simulink model "buckcomverter+battery"  (R2020a)
settings: Solver=VariableStepAuto  StartTime=0.0  StopTime=5  RelTol=1e-3
undefined symbols (not defined in the file): Acid, Down, Lead, Up
libraries: powerlib x9, electricdrivelib x1, eePwmGenerator x1
settings Model: Creator=Asus  LastModifiedBy=asus
settings DataIOCC: ReturnWorkspaceOutputs=off
settings DebuggingCC: ArithmeticOperatorsInVariantConditions=warning
settings SFSimCC: CustomCodeUndefinedFunction=UseInterfaceOnly

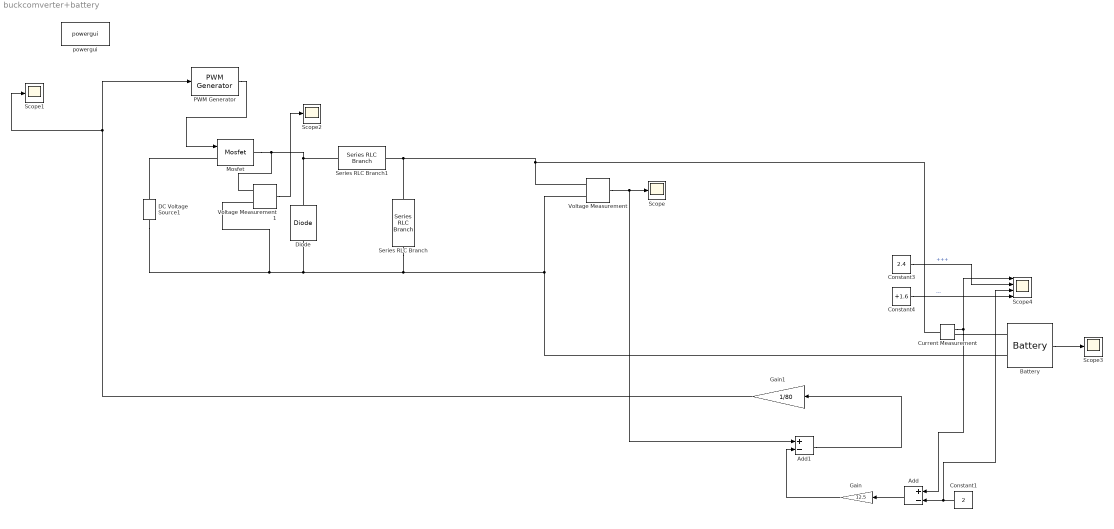
== system buckcomverter+battery ==
  Add : Sum  Inputs=+-
  Add1 : Sum  Inputs=+-
  Battery : electricdrivelib/Extra Sources/Battery  BatType=Lead-Acid  ShowTempParam=off  ThermalPreset=no  ShowAgeParam=off  NomV=24  NomQ=13  SOC=50  Batt_Tr=0.000001  PresetModel=on  MaxQ=13.5417  MinV=18  FullV=26.1316  Dis_rate=2.6  R=0.018462  Normal_OP=4.0336  expZone="[24.4342    0.0433333]"  current=[6.5 13 32.5]  Units=Time  Tci=20  NomT=20  T2=-30  MaxQ2=4.8  FullV2=7.1  Normal_OP2=5.655  expZone2="[6.58           1]"  Rca=0.6  ti=2000  Dp=0  Neq0=0  Tsim=1e6  Ta1=25  Qeol=5.4*0.9  Reol=0.013333*1.2  Char_age=[2.3478, 3]  Dis_age=[2.3478, 10]  N1=1500  N2=10500  N3=1000  N4=1400  Ta2=45  N5=950
  Constant1 : Constant  Value=2
  Constant3 : Constant  Value=2.4
  Constant4 : Constant  Value=+1.6
  Current Measurement : powerlib/Measurements/Current Measurement  PhasorSimulation=off  OutputType=Complex  PSBequivalent=0
  DC Voltage Source1 : powerlib/Electrical Sources/DC Voltage Source  Amplitude=80  Measurements=None
  Diode : powerlib/Power Electronics/Diode  Ron=0.001  Lon=0  Vf=0.8  IC=0  UseSnubber=0  Rs=500  Cs=250e-9  Measurements=off
  Gain : Gain  Gain=12.5
  Gain1 : Gain  Gain=1/80
  Mosfet : powerlib/Power Electronics/Mosfet  Ron=0.1  Lon=0  Rd=0.01  Vfd=0  IC=0  Rs=1e5  Cs=inf  Measurements=off
  PWM Generator : eePwmGenerator/PWM Generator  CarrCount=Up-Down  Tper=1e-4  Ts=5e-6
  Scope{,1..3} (4 alike) : Scope
  Scope4 : Scope  NumInputPorts=4
  Series RLC Branch : powerlib/Elements/Series RLC Branch  LConnTagsString=__new0  RConnTagsString=__new0  BranchType=C  Resistance=1  Inductance=1e-3  SetiL0=off  InitialCurrent=0  Capacitance=3e-4  Setx0=on  InitialVoltage=24.1  Measurements=None
  Series RLC Branch1 : powerlib/Elements/Series RLC Branch  LConnTagsString=__new0  RConnTagsString=__new0  BranchType=L  Resistance=1  Inductance=3.68e-3  SetiL0=off  InitialCurrent=0  Capacitance=1e-6  Setx0=off  InitialVoltage=0  Measurements=None
  Voltage Measurement : powerlib/Measurements/Voltage Measurement  PhasorSimulation=off  OutputType=Complex  PSBequivalent=0
  Voltage Measurement1 : powerlib/Measurements/Voltage Measurement  PhasorSimulation=off  OutputType=Complex  PSBequivalent=0
  powergui : powerlib/powergui  Priority=1  SimulationMode=Continuous  SampleTime=50e-6  frequency=60  Iterations=50  frequencyindice=0  Pbase=100e6  ErrMax=1e-4  UnitsV=kV  UnitsW=MW  buscounter=0  FunctionMessages=off  echomessages=off  EnableUseOfTLC=off  CurrentSourceSwitches=off  DisableSnubberDevices=off  DisableRonSwitches=off  DisableVfSwitches=off  DisplayEquations=off  AutomaticDiscreteSolvers=off  SolverType=Tustin/Backward Euler (TBE)  Interpol=off  ExternalGateDelay=off  methode=off  Ts=100  x0status=blocks  SPID=on  SwTol=0  HookPort=off  NonlinearTolerance=1e-4  nMaxIteration=100  ContinueOnMaxIteration=off  RestoreLinks=warning  ResistiveCurrentMeasurement=off  Frange=[0:2:500]  Ylog=off  Xlog=on  ShowGrid=off  save=off  variable=ZData  structure=0  ZoomFFT=off  StartTime=0.0  cycles=1  DisplayStyle=1  fundamental=60  FreqAxis=off  MaxFrequency=1000  frequencyindicesteady=1  RmsSteady=1  display=off
  wires:
  PWM Generator/1 -> Mosfet/1
  Voltage Measurement/1 -> Add1/1, Scope/1
  Voltage Measurement1/1 -> Scope2/1
  Constant3/1 -> Scope4/2  "+++"
  Gain1/1 -> Scope1/1, PWM Generator/1
  Gain/1 -> Add1/2
  Current Measurement/1 -> Scope4/1, Add/1
  Add/1 -> Gain/1
  Constant1/1 -> Scope4/3, Add/2
  Add1/1 -> Gain1/1
  Constant4/1 -> Scope4/4  "---"
  Battery/1 -> Scope3/1
  connections:
  DC Voltage Source1/RConn1 -- Mosfet/LConn1
  Mosfet/RConn1 -- Voltage Measurement1/LConn1 -- Series RLC Branch1/LConn1 -- Diode/RConn1
  DC Voltage Source1/LConn1 -- Voltage Measurement1/LConn2 -- Voltage Measurement/LConn2 -- Battery/LConn2 -- Series RLC Branch/RConn1 -- Diode/LConn1
  Voltage Measurement/LConn1 -- Current Measurement/LConn1 -- Series RLC Branch/LConn1 -- Series RLC Branch1/RConn1
  Current Measurement/RConn1 -- Battery/LConn1
